simulink model "second_order_system"  (R2021a)
settings: Solver=VariableStepAuto  StartTime=0.0  StopTime=10.0  RelTol=1e-3
values from neighbouring files (symbols this model uses):
  alpha = 1    [second_order_system_m.m]
  wn = 10    [second_order_system_m.m]
  zeta = 0.2    [second_order_system_m.m]
settings Model: Creator=jun  LastModifiedBy=jun

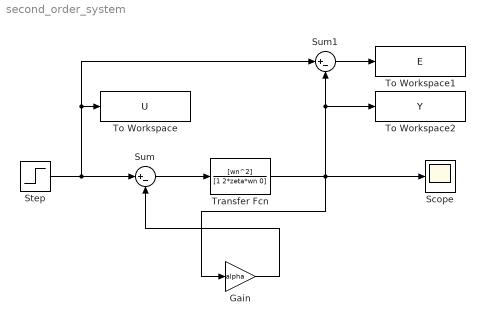
== system second_order_system ==
  Gain : Gain  Gain=alpha
  Scope : Scope
  Step : Step  SampleTime=0
  Sum : Sum  Inputs=|+-
  Sum1 : Sum  Inputs=|+-
  To Workspace : ToWorkspace  VariableName=U  SaveFormat=Timeseries  SampleTime=-1
  To Workspace1 : ToWorkspace  VariableName=E  SaveFormat=Timeseries  SampleTime=-1
  To Workspace2 : ToWorkspace  VariableName=Y  SaveFormat=Timeseries  SampleTime=-1
  Transfer Fcn : TransferFcn  Numerator=[wn^2]  Denominator=[1 2*zeta*wn 0]
  wires:
  Step/1 -> Sum1/1, To Workspace/1, Sum/1
  Sum/1 -> Transfer Fcn/1
  Transfer Fcn/1 -> Gain/1, To Workspace2/1, Sum1/2, Scope/1
  Sum1/1 -> To Workspace1/1
  Gain/1 -> Sum/2
